simulink model "phase_magrin_sine"  (R2022a)
settings: Solver=VariableStepAuto  StartTime=0.0  StopTime=25  MaxStep=0.01  RelTol=1e-3
settings Model: PacingRate=0.500000  Creator=oyxl  LastModifiedBy=oyxl

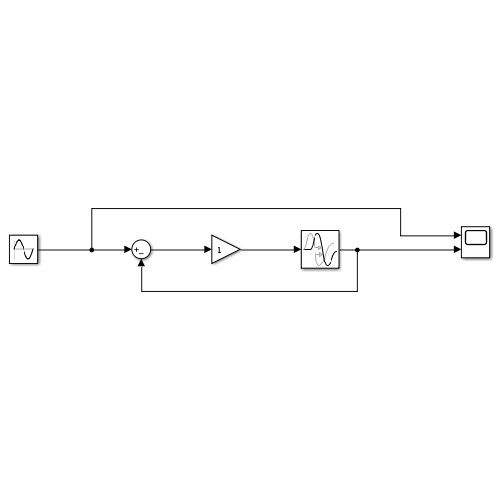
[thumbnail: Simulink's stored preview of the top-level diagram]
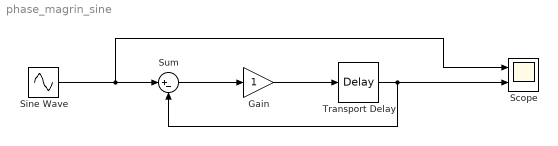
== system phase_magrin_sine ==
  Gain : Gain
  Scope : Scope  NumInputPorts=2
  Sine Wave : Sin  Frequency=2*pi  SampleTime=0
  Sum : Sum  Inputs=|+-
  Transport Delay : TransportDelay  DelayTime=0.5
  wires:
  Transport Delay/1 -> Sum/2, Scope/2
  Sum/1 -> Gain/1
  Gain/1 -> Transport Delay/1
  Sine Wave/1 -> Scope/1, Sum/1
